simulink model "Reverse_01"  (R2018b)
settings: Solver=VariableStepAuto  StartTime=0.0  StopTime=60  RelTol=1e-3
libraries: simulink x2
settings Model: Creator=ali  LastModifiedBy=ali

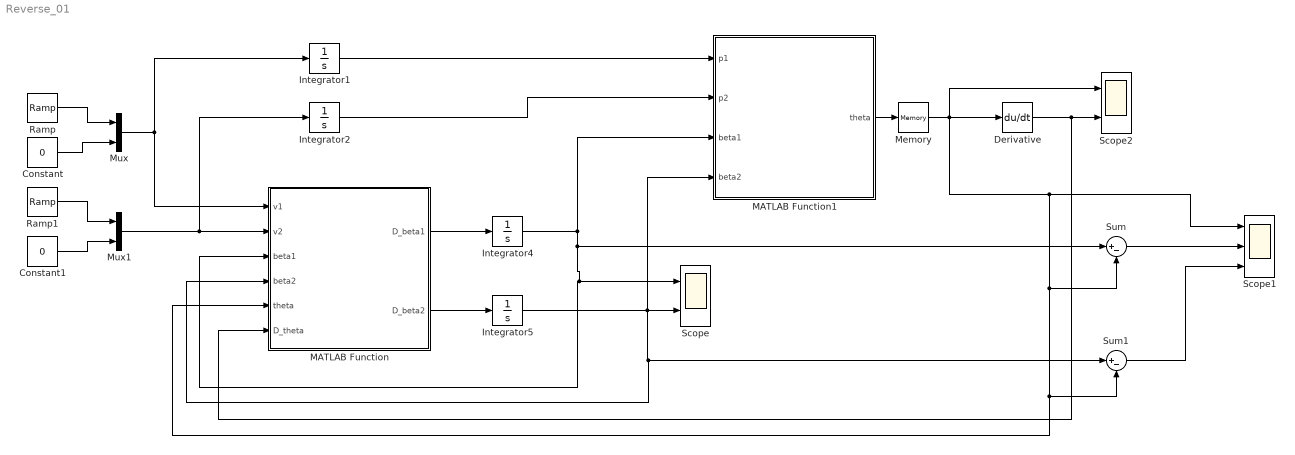
== system Reverse_01 ==
  Constant : Constant  Value=0
  Constant1 : Constant  Value=0
  Derivative : Derivative
  Integrator1 : Integrator  InitialCondition=[0;0]
  Integrator2 : Integrator  InitialCondition=[0;0]
  Integrator4 : Integrator  InitialCondition=pi/4
  Integrator5 : Integrator  InitialCondition=pi/4
  MATLAB Function : MATLAB Function  TreatAsAtomicUnit=on
  MATLAB Function1 : MATLAB Function  TreatAsAtomicUnit=on
  Memory : Memory
  Mux : Mux  Inputs=2
  Mux1 : Mux  Inputs=2
  Ramp : simulink/Sources/Ramp  slope=1  start=10  InitialOutput=0
  Ramp1 : simulink/Sources/Ramp  slope=1  start=10  InitialOutput=0
  Scope : Scope  NumInputPorts=2
  Scope1 : Scope  NumInputPorts=3
  Scope2 : Scope  NumInputPorts=2
  Sum : Sum  Inputs=|+-
  Sum1 : Sum  Inputs=|+-
  wires:
  MATLAB Function/2(D_beta2) -> Integrator5/1
  MATLAB Function/1(D_beta1) -> Integrator4/1
  Ramp/1 -> Mux/1
  Ramp1/1 -> Mux1/1
  Constant/1 -> Mux/2
  Constant1/1 -> Mux1/2
  Mux/1 -> Integrator1/1, MATLAB Function/1(v1)
  Mux1/1 -> Integrator2/1, MATLAB Function/2(v2)
  MATLAB Function1/1(theta) -> Memory/1
  Derivative/1 -> MATLAB Function/6(D_theta), Scope2/2
  Integrator1/1 -> MATLAB Function1/1(p1)
  Integrator2/1 -> MATLAB Function1/2(p2)
  Integrator4/1 -> Sum/1, MATLAB Function/3(beta1), Scope/1, MATLAB Function1/3(beta1)
  Integrator5/1 -> MATLAB Function1/4(beta2), Scope/2, MATLAB Function/4(beta2), Sum1/1
  Sum/1 -> Scope1/2
  Sum1/1 -> Scope1/3
  Memory/1 -> Scope1/1, Sum/2, MATLAB Function/5(theta), Sum1/2, Scope2/1, Derivative/1

== matlab function Reverse_01/MATLAB Function1 ==
  data: p1 input; theta output; p2 input; beta1 input; beta2 input
function theta = fcn(p1,p2,beta1,beta2)

l = 1;

theta = atan( (p1(2)-p2(2)-l*(sin(beta1)+sin(beta2))) / (p1(1)-p2(1)-l*(cos(beta1)+cos(beta2))) ); 

end

== matlab function Reverse_01/MATLAB Function ==
  data: v1 input; D_beta1 output; v2 input; beta1 input; beta2 input; theta input; D_theta input; D_beta2 output
function [D_beta1,D_beta2] = fcn(v1,v2,beta1,beta2,theta,D_theta)

l = 1;
d = 1;

F = [v1(1)-v2(1);v1(2)-v2(2)];

A = [-l*sin(beta1) -1*sin(beta2);
    l*cos(beta1) l*cos(beta2)];

B = [-2*d*D_theta*sin(theta);2*d*D_theta*cos(theta)];

DX = ((A'*A)^(-1)) * A' * (F-B);

D_beta1 = DX(1);
D_beta2 = DX(2);

end
